simulink library "CELCmgrLogicLib"  (R2017b)
settings: Solver=ode45  StartTime=0.0  StopTime=10.0  RelTol=1e-3  EnableMultiTasking=on
undefined symbols (not defined in the file): CELCmgr_EgyClimaAllwdFac, CELCmgr_EgyCnsAllwdForClimaMax, CELCmgr_TclimaMax, CELCmgr_TEgyChkTime_5min
settings Model: Creator=uidp6624  LastModifiedBy=Xiao Tao
settings DataIOCC: LimitDataPoints=on
settings OptimizationCC: LifeSpan=inf
settings DebuggingCC: AllowSymbolicDim=off  SFUnexpectedBacktrackingDiag=warning  SFNoUnconditionalDefaultTransitionDiag=warning  SFExecutionAtInitializationDiag=none
settings CodeAppCC: StateflowObjectComments=on
settings GRTTargetCC: TargetLangStandard=C89/C90 (ANSI)  GeneratePreprocessorConditionals=Disable all
settings ConfigComp: CovMetricSettings=dw  CovHtmlReporting=on  CovSaveCumulativeToWorkspaceVar=on  CovSaveSingleToWorkspaceVar=on  CovExternalEMLEnable=off

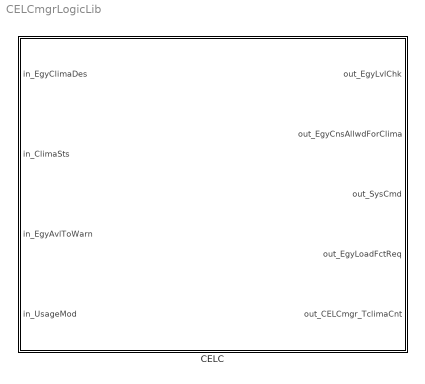
== system CELCmgrLogicLib ==
  CELC : Stateflow chart  TreatAsAtomicUnit=on

== stateflow chart CELCmgrLogicLib/CELC ==
  state CELC_ACTUATOR_OFF
    en,du:
    InactiveUsageMode();
  state InactiveUsageMode [function]
    (default) -> (junction 199) : {out_CELCmgr_TclimaCnt = 0;
        | /*Stop actuator work*/
        | out_SysCmd = 0;
        | /*Stop energy level check*/
        | out_EgyLvlChk = 0;}
    (junction 199) -> (junction 130) : /*Climate finished working*/
        | [in_ClimaSts != 0]
    (junction 130) -> (junction 145) : /*Inactive energy load usage mode*/
        | {out_EgyLoadFctReq = 0;}
  state CELC_ACTUATOR_ON
    en,du:
    /*Start actuator working*/
    out_SysCmd = 1;
  state SystemEgyCalc [function]
    (default) -> (junction 173) : {out_EgyCnsAllwdForClima = in_EgyAvlToWarn * 12 * CELCmgr_EgyClimaAllwdFac;}
    (junction 173) -> (junction 175) : [out_EgyCnsAllwdForClima > CELCmgr_EgyCnsAllwdForClimaMax]
    (junction 175) -> (junction 174) : {out_EgyCnsAllwdForClima = CELCmgr_EgyCnsAllwdForClimaMax;}
  state CELC_EGY_CHECK
    en:
    out_CELCmgr_TclimaCnt++;
    en,du:
    out_EgyLvlChk =1;
  state CELC_SYS_EGY_CALC
    en,du:
    /*REQPROD_216022*/
    SystemEgyCalc();
  state CELC_ACTV_USG_MODE
    en,du:
    /*Disable energy level check*/
    out_EgyLvlChk = 0;
    /*Active energy load usage mode*/
    out_EgyLoadFctReq = 1;
  (default) -> CELC_ACTUATOR_OFF
  (junction 190) -> CELC_ACTUATOR_OFF
  (junction 182) -> CELC_ACTUATOR_OFF
  CELC_ACTUATOR_ON -> (junction 190) [order 2] : /*REQPROD_216020
      | Usage mode is abandoned or no energy consuption request
      | or clima worked more than 60min*/
      | [(in_UsageMod == 0)...
      | ||(in_EgyClimaDes == 0)...
      | || (out_CELCmgr_TclimaCnt  >= CELCmgr_TclimaMax+1)]
  CELC_SYS_EGY_CALC -> (junction 182) [order 2]
  CELC_ACTUATOR_OFF -> CELC_EGY_CHECK : /*REQPROD_216018
      | Usage mode is  abandoned and reveive energy consumption request*/
      | [(in_UsageMod == 0)...
      | && (in_EgyClimaDes > 0)]
  CELC_ACTUATOR_ON -> CELC_EGY_CHECK [order 1] : /*REQPROD_216018
      | Send check engergy level request every 5min */
      | [after(CELCmgr_TEgyChkTime_5min,tick)]
  CELC_EGY_CHECK -> CELC_SYS_EGY_CALC : [in_EgyAvlToWarn > 0]
  CELC_SYS_EGY_CALC -> (junction 185) [order 1] : /*Climate allowed to work*/
      | [in_ClimaSts == 0]
  (junction 186) -> CELC_ACTUATOR_ON
  CELC_ACTV_USG_MODE -> (junction 186) : /*Usage mode is not abandoned*/
      | [in_UsageMod != 0]
  (junction 185) -> CELC_ACTV_USG_MODE
  data: in_EgyClimaDes input uint16; in_ClimaSts input uint8; out_EgyLvlChk output uint8; in_EgyAvlToWarn input uint16; CELCmgr_TclimaMax parameter uint8; out_EgyCnsAllwdForClima output uint16 =0; in_UsageMod input uint8; out_SysCmd output uint8; out_EgyLoadFctReq output uint8; CELCmgr_TEgyChkTime_5min parameter uint16; CELCmgr_EgyClimaAllwdFac parameter uint8; out_CELCmgr_TclimaCnt output uint8; CELCmgr_EgyCnsAllwdForClimaMax parameter uint8
